simulink model "dspaudiosrc"  (Simulink 8.3)
settings: Solver=FixedStepDiscrete  SolverMode=SingleTasking  StartTime=0.0  StopTime=inf  RelTol=1e-3
model workspace (MATLAB code in the model file):
  | load dspaudiosrc
libraries: dspsrcs4 x1, dspmlti4 x1, dspmisc x1
settings Model: Creator=The MathWorks Inc.  ExtModeAutoUpdateStatusClock=off
settings DataIOCC: SaveOutput=off  SignalLogging=off  SaveTime=off
settings OptimizationCC: InlineParams=on  ExpressionDepthLimit=2147483647  InitFltsAndDblsToZero=on
settings DebuggingCC: SignalResolutionControl=TryResolveAllWithWarning  SolverPrmCheckMsg=none  MultiTaskDSMMsg=warning  MultiTaskCondExecSysMsg=none  ParameterPrecisionLossMsg=none  FcnCallInpInsideContextMsg=UseLocalSettings
settings HardwareCC: ProdHWDeviceType=ASIC/FPGA  TargetHWDeviceType=32-bit Generic  ProdEqTarget=off
settings RTWCC: IncludeERTFirstTime=on

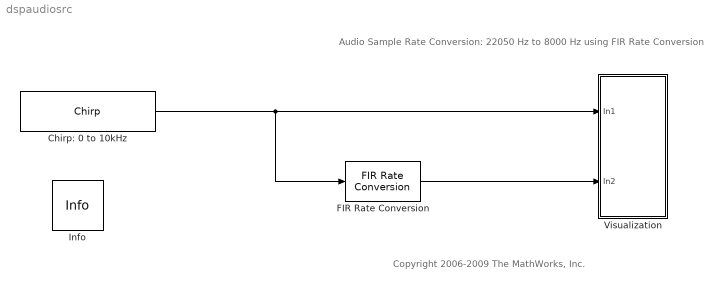
== system dspaudiosrc ==
  note: Audio Sample Rate Conversion:
      | 22050 Hz to 8000 Hz using FIR Rate Conversion
  note: Copyright 2006-2009 The MathWorks, Inc.
  Chirp: 0 to 10kHz : dspsrcs4/Chirp  sweep=Linear  mode=Bidirectional  f0=0  f1=10000  t1=10  Tsweep=10  phase=0  Ts=1/22050  spf=441  datatype=Double
  FIR Rate Conversion : dspmlti4/FIR Rate Conversion  Tag=BlockMethodSubSystem  L=160  h=b  M=441  firstCoeffMode=Specify word length  firstCoeffWordLength=16  firstCoeffFracLength=0  firstCoeffDataTypeStr=fixdt(1,16)  firstCoeffLastDataTypeStr=fixdt(1,16)  firstCoeffMin=[]  firstCoeffMax=[]  outputMode=Binary point scaling  outputWordLength=16  outputFracLength=15  outputDataTypeStr=fixdt(1,16,15)  outputLastDataTypeStr=fixdt(1,16,15)  outputMin=[]  outputMax=[]  accumMode=Binary point scaling  accumWordLength=32  accumFracLength=30  accumDataTypeStr=fixdt(1,32,30)  accumLastDataTypeStr=fixdt(1,32,30)  roundingMode=Nearest  overflowMode=on  FilterSource=Specify via dialog  FilterObject=Hm_firsrc
  Info : dspmisc/Info  SystemSampleTime=-1
  Visualization : Subsystem
      mask Display: disp('SCOPES')
  wires:
  Chirp: 0 to 10kHz/1 -> Visualization/1(In1), FIR Rate Conversion/1
  FIR Rate Conversion/1 -> Visualization/2(In2)

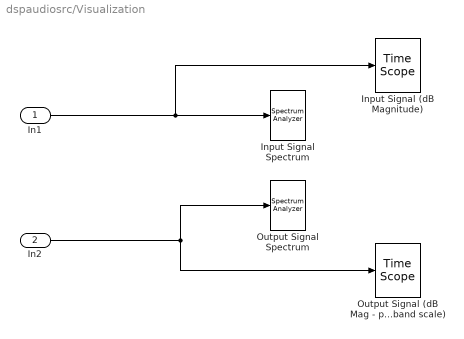
== system dspaudiosrc/Visualization ==
  In1 : Inport
  In2 : Inport  Port=2
  Input Signal (dB Magnitude) : TimeScope  DefaultConfigurationName=spbscopes.TimeScopeBlockCfg  ScopeSpecification=DataTag0
  Input Signal Spectrum : SpectrumAnalyzer  ScopeSpecification=DataTag1
  Output Signal (dB Mag - passband scale) : TimeScope  DefaultConfigurationName=spbscopes.TimeScopeBlockCfg  ScopeSpecification=DataTag2
  Output Signal Spectrum : SpectrumAnalyzer  ScopeSpecification=DataTag3
  wires:
  In1/1 -> Input Signal Spectrum/1, Input Signal (dB Magnitude)/1
  In2/1 -> Output Signal Spectrum/1, Output Signal (dB Mag - passband scale)/1
